simulink model "Suspension"  (R2018b)
settings: Solver=VariableStepAuto  StartTime=0.0  StopTime=10.0  RelTol=1e-3
values from neighbouring files (symbols this model uses):
  Ks = 2e4    (= 20000)    [CarQuarterParam.m]
undefined symbols (not defined in the file or in its folder): Cs
settings Model: Creator=Reece Bell  LastModifiedBy=Reece Bell

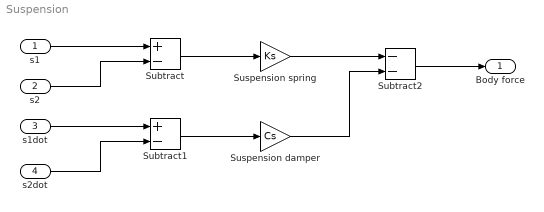
== system Suspension ==
  s1 : Inport
  s2 : Inport  Port=2
  "s1dot " : Inport  Port=3
  s2dot : Inport  Port=4
  Subtract : Sum  Inputs=+-
  Subtract1 : Sum  Inputs=+-
  Subtract2 : Sum  Inputs=--
  Suspension damper : Gain  Gain=Cs
  Suspension spring : Gain  Gain=Ks
  Body force : Outport
  wires:
  s1/1 -> Subtract/1
  s2/1 -> Subtract/2
  "s1dot "/1 -> Subtract1/1
  s2dot/1 -> Subtract1/2
  Subtract/1 -> Suspension spring/1
  Subtract1/1 -> Suspension damper/1
  Suspension spring/1 -> Subtract2/1
  Suspension damper/1 -> Subtract2/2
  Subtract2/1 -> Body force/1
